simulink model "USBamp_offline"  (R2015a)
settings: Solver=ode45  StartTime=0.0  StopTime=Inf  RelTol=1e-3
undefined symbols (not defined in the file or in its folder): currentCFG_USBamp_offline_UB, UB
libraries: dspbuff3 x2, Tools x1, gtecHighspeedLib x1, gUSBamplib x1
settings Model: Creator=Co  LastModifiedBy=Co
settings OptimizationCC: BlockReduction=off

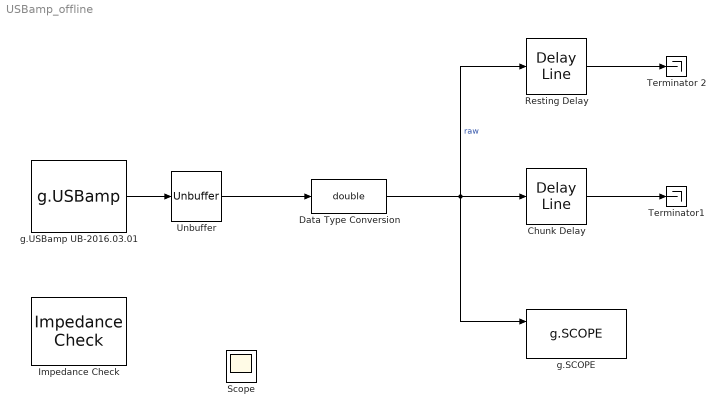
== system USBamp_offline ==
  Chunk Delay : dspbuff3/Delay Line  siz=512  ic=0  directfeed=off  enable_output=off  hold_output=off  TreatMby1Signals=One channel
  Data Type Conversion : DataTypeConversion  OutDataTypeStr=double
  Impedance Check : Tools/Impedance Check
  Resting Delay : dspbuff3/Delay Line  siz=512  ic=0  directfeed=off  enable_output=off  hold_output=off  TreatMby1Signals=One channel
  Scope : Scope
  Terminator 2 : Terminator
  Terminator1 : Terminator
  Unbuffer : Unbuffer  SampleBasedProcessing=Same as frame based
  g.SCOPE : gtecHighspeedLib/g.SCOPE
  g.USBamp UB-2016.03.01 : gUSBamplib/g.USBamp  cfg=currentCFG_USBamp_offline_UB-2016.03.01.cfg  snr=UB-2016.03.01
  wires:
  g.USBamp UB-2016.03.01/1 -> Unbuffer/1
  Unbuffer/1 -> Data Type Conversion/1
  Data Type Conversion/1 -> Resting Delay/1, Chunk Delay/1, g.SCOPE/1  "raw"
  Resting Delay/1 -> Terminator 2/1
  Chunk Delay/1 -> Terminator1/1
